simulink model "Quadcopter_v4_full"  (R2021a)
settings: Solver=ode4  StartTime=0.0  StopTime=87  FixedStep=0.001  RelTol=1e-6
values from neighbouring files (symbols this model uses):
  mean_wind = [2.72 , 1.75, -0.006]    [main_run.m]    (also in main_run_5_1.m; param_est.m = [2.72 , 1.75, .006])
  q = X(7:10)    [EKF_without_wind.m]
  r = linspace(floor(nr*0.01)/nr,1,nr)    [main_run.m]    (also in main_run_5_1.m)
  w1 = w(1)    [EKF_without_wind.m]
  x0 = [0,0,0,1,0,0,0,-P.mean_wind,0,0,0]    [main_run.m]    (also in main_run_5_1.m)
  xref = [1,1,-8,1,0,0,0,-P.mean_wind]    [main_run.m]    (also in main_run_5_1.m)
undefined symbols (not defined in the file or in its folder): HDBK, MIL, Moderate, P, u1, v1
libraries: simulink x1, aerolibwind2 x1
(part 5 of 5)

== matlab function Quadcopter_v4_full/Rotor Dynamics /SBEMT/Simplified BEMT ==
  data: V_rb input; Y output; rpm input; P parameter
function Y  = simplified_BEMT(V_rb,rpm,P)
%simplified BEMT model Summary of this function goes here
%   Detailed explanation goes here
% q_i  = X(4:7);
% vr_i = X(8:10);
% 
% eul = quat2eul(q_i')';
% eul([1 3]) = eul([3 1]);
% roll = eul(1);
% pitch = eul(2);
% yaw = eul(3);
% x_axis=[1;0;0];y_axis=[0;1;0];z_axis=[0;0;1]; 
% R_ib = expm(hat(z_axis)*yaw)*expm(hat(y_axis)*pitch)*expm(hat(x_axis)*roll);
% vr_b = R_ib'*vr_i;

% Asma: So Vr_b here is the exact input going into actual BMET optimization
% block, it is already calculated so no need for additional calculation
vr_b = V_rb;
rpm =mean(rpm)/16000;
%%
weights = P.weights;
n_lay_neu = P.n_lay_neu;

features = 4;
weights1 = cell(1,length(n_lay_neu));
for i=1:1:length(n_lay_neu)
    if i==1 
        index_input = features+1;                %+1 means add the bias row
        index_output = n_lay_neu(i);
        weights1{i} = weights(1:index_input,1:index_output);
    else
        index_input_pre = index_input;
        index_input = index_input_pre + n_lay_neu(i-1) + 1;
        index_output = n_lay_neu(i);
        weights1{i} = weights(index_input_pre+1:index_input,1:index_output);
    end 
end
%% 
% In order to require the code generator's requirement, we declare the
% thrust_forward_NN as the extrinsic function
coder.extrinsic('thrust_forward_NN'); 
Y = zeros(1);
Y = thrust_forward_NN([vr_b' rpm],weights1,n_lay_neu);%normalize the rpm(16000)
Y = 4*Y;
end

== matlab function Quadcopter_v4_full/wind/Dryden Wind/Input/DCM//rotation matrix ==
  data: x input; R output
function R = fcn(x)
phi = x(7);theta = x(8);psi = x(9);
% rotation from inertial frame to body frame
R = [1, 0, 0;0, cos(phi), sin(phi);0, -sin(phi), cos(phi)]*[cos(theta),...
    0, -sin(theta);0, 1, 0;sin(theta), 0, cos(theta)]*[cos(psi),...
    sin(psi), 0;-sin(psi), cos(psi), 0;0, 0, 1];
R = inv(R);
end

== matlab function Quadcopter_v4_full/wind/Dryden Wind/Input/MATLAB Function ==
  data: wind input; V output; vel input
function V = fcn(wind,vel)
%#codegen
V = norm(wind - vel);
end

== matlab function Quadcopter_v4_full/wind/Dryden Wind/Input1/DCM//rotation matrix ==
  data: x input; y output
function y = fcn(x)
phi = x(7);theta = x(8);psi = x(9);
% rotation from inertial frame to body frame
R = [1, 0, 0;0, cos(phi), sin(phi);0, -sin(phi), cos(phi)]*[cos(theta),...
    0, -sin(theta);0, 1, 0;sin(theta), 0, cos(theta)]*[cos(psi),...
    sin(psi), 0;-sin(psi), cos(psi), 0;0, 0, 1];
R = inv(R);
y = R;

== matlab function Quadcopter_v4_full/wind/Dryden Wind/Input1/MATLAB Function ==
  data: wind input; V output; vel input; P parameter
function V = fcn(wind,vel,P)
%#codegen
V = norm(wind - vel);
end

== matlab function Quadcopter_v4_full/wind/Dryden Wind/Select velocities/Merge Subsystems/convert to inertial frame ==
  data: ug input; ugw output; vg input; wg input; dcm input; vgw output; wgw output
function [ugw,vgw,wgw] = fcn(ug,vg,wg,dcm)
%#codegen
u = dcm*[ug;vg;wg];
ugw = u(1);
vgw = u(2);
wgw = u(3);

== matlab function Quadcopter_v4_full/quadcopter/MATLAB Function ==
  settings: updateMethod=DISCRETE
  data: X input; U input; wind input; t_c input; X_dot output; P parameter; wdot output; R output
function [X_dot,wdot,R]  = quad_model(X,U,wind,t_c,P)

%#codegen
%References: Dynamics using Quaternion for full-state feedback control
%adapted from "Onboard State Dependent LQR for Agile Quadrotors"
%see "AIAA paper draft for full model"

%parameters
m = P.m;
g = P.g;
rho = P.rho;

Ix = P.Ix;
Iy = P.Iy;
Iz = P.Iz;
J=[Ix , 0 , 0;
    0 , Iy , 0;
    0 , 0  , Iz];

D   = P.D;
%states
% p_i = X(1:3);
q_i  = X(4:7);
% hao 10/27/2021 normalize the unit quaternion
q_i=q_i/norm(q_i);

v_i = X(8:10);
w_b = X(11:13);
% disp(w_b)


%inputs

F_c = [0;0;U(1)];
tau=[U(2);
     U(3);
     U(4)];
 
%% system dynamics with drag in WORLD FRAME
%HAO: what is this?
% wind(3)=-wind(3);%wind from CFD data is positive upward

R=quater_rot(q_i);

% eul = quat2eul(q_i')';
% eul([1 3]) = eul([3 1]);
% roll = eul(1);
% pitch = eul(2);
% yaw = eul(3);
% x_axis=[1;0;0];y_axis=[0;1;0];z_axis=[0;0;1]; 
% R = expm(hat(z_axis)*yaw)*expm(hat(y_axis)*pitch)*expm(hat(x_axis)*roll);

% R = quat2R(q_i');



dp = v_i+wind;
dq = 0.5*quater_mult(q_i)*[0;w_b];
% dv = ([0;0;g] - R*F_c-norm(v_i)*R*D*R'*v_i)/m;
% dv = ([0;0;m*g] - R*F_c-0.5*rho*norm(v_i)*R*D*R'*v_i)/m; %10/20/2021 Hao
f_vr=-(1/2)*rho*D*norm(R'*v_i)*(R'*v_i);
dv = ([0;0;m*g] - R*F_c + R*f_vr)/m;


dwb = J\(tau-cross(w_b,(J*w_b)));

X_dot=[dp ; dq ; dv ; dwb]';
wdot=dwb;


end


function R = quater_rot(q)

w = q(1);
x = q(2);
y = q(3);
z = q(4);

Q = [w -x -y -z;...
     x w -z y;...
     y z w -x;...
     z -y x w];

Qc =[w -x -y -z;...
     x w z -y;...
     y -z w x;...
     z y -x w];
t = Qc'*Q;
R = t(2:4,2:4);
end


function Q = quater_mult(q)

w = q(1);
x = q(2);
y = q(3);
z = q(4);

Q = [w -x -y -z;...
     x w -z y;...
     y z w -x;...
     z -y x w];

end

== matlab function Quadcopter_v4_full/Controller /High Level Controller/trajectory/MATLAB Function ==
  data: t input; xdes output; P parameter
function xdes = getref(t,P)

% This function tracks time and match nominal trajectory at next nearest
% time
% Input:
% nomTraj is the nominal trajectory with t
% 
nomTraj = P.nomTraj;
idxA = find(nomTraj(:,1)>=t);
idx=idxA(1);
xdes=nomTraj(idx,2:end);

== matlab function Quadcopter_v4_full/MATLAB Function ==
  data: u input; omega output; P parameter
function omega = motor_omega(u, P)

%omega = u;
%prevent negative F because the calculation only need the value of fc
% if u(1)<0
%     u(1)=-u(1);
% end
%prevent too high of a moment
for i=2:3
    if u(i)>.15*u(1)
        u(i)=.15*u(1);    %why?
    end
end

L = P.l;
b= P.b;
k = P.k;
% 
A = [b b b b;
    0 L*b 0 -L*b;
    L*b 0 -L*b 0;   %from BMET Code 
    k -k k -k];  %

% A = [b b b b;
%     0 -L*b 0 L*b;
%     -L*b 0 L*b 0;   %from source Trajectory tracking control design with command-filtered compensation for a quadrotor
%     -k k -k k]; 


% A = [b b b b;
%     0 -L*b 0 L*b;
%     L*b 0 -L*b 0;   %Tryng my ways
%     k -k k -k];  %

%R matrix just changes which direction the 'front' of the quad is
%without it,quadcopter would be '+' type;with it,quadcopter would be 'x' type
% offset = pi/4;
% R = [1 0 0 0;
%     0 cos(offset) -sin(offset) 0;
%     0 sin(offset) cos(offset) 0;
%     0 0 0 1];
% omega_squared = pinv(A)*R*u; %pinv-Pseudoinverse

omega_squared = pinv(A)*u'; %pinv-Pseudoinverse

for i=1:4
    if omega_squared(i) < 0
        omega_squared(i) = 0;
    end
end

omega = sqrt(omega_squared);
%hao 20/27/2021 set limit to the rpm
% for i=1:4
%     if omega(i) >16000
%         omega(i) = 16000;
%     end
% end 

end

== matlab function Quadcopter_v4_full/Rotor Dynamics /BEMT(from datagen)/MATLAB Function1 ==
  settings: updateMethod=DISCRETE
  data: rpm_guesses input; V_rel_b input; U_final output; P parameter; geometry data_store_memory
function U_final  = FWF_BEMT_adjustment(rpm_guesses,V_rel_b, P)


% governing equations
% governing equations

% T=T1+T2+T3+T4 ;
% TA1=l*(T4-T2) ;   roll positive right wing down
% TA2=l*(T1-T3) ;   pitch up positive
% TA3=ta1+ta2+ta3+ta4 ;

% it looks like in atitude control output of the functin should be pitch
% down positive
% Not Related with LQR CONTROL ASMA*

%%
% predefining vriables for Codegen

k = P.k;
b = P.b;
l = P.l;
T_final=0;
Tau_initial=zeros(3,1);
Tau_final=zeros(3,1);
T2=zeros(4,1);
pow=zeros(4,1);

TA=zeros(3,1);
TA1=zeros(4,1);
TA2=zeros(4,1);
TA3=zeros(4,1);
ta1=zeros(4,1);
ta2=zeros(4,1);
ta3=zeros(4,1);

RPM2=single(zeros(4,1));
RPM=zeros(4,1);

T = b * rpm_guesses.^2;       % requested thrust from rotor r
Tau = k * rpm_guesses.^2;     % requested torques from rotor r

%%for calculation transforming all information into vector form
% rel_speed = V_info(1);
% heading = deg2rad(V_info(2));
% v_rel_z = V_info(3);
% 
% v_rel_x = rel_speed*cos(heading);
% v_rel_y = rel_speed*sin(heading);
% 
% V_rel_b = [v_rel_x,v_rel_y,v_rel_z];


for i=1:4
    % optimization to find optimum rpm where both momentum annd blade element theories match
    
    subfcn2 = @(rpm) try1(rpm,V_rel_b,T(i));
    
    rpm=golden_search(0,17000,subfcn2); %limits of RPM, checked that the higher limit goes beyond 25000 so chaging from 100 16000
    
    [~,roll,pitch,yaw,~,lambda1]=try1(rpm,V_rel_b,T(i));
    
    % rpm to rad/second
    RPM(i)=rpm ;%*2*pi/60; NO NEED ASMA
    
    % torques of a rotor - rotor 1 is the leading edge rotor,left
    % number 2, right number 4, aft number, 1 and 3 ccw. 2 and 4 cw.
    
    heading=atan(V_rel_b(2)/(V_rel_b(1)+0.000001));
    ta1(i) = roll * cos(heading) * (-1)^(i+1) - pitch * sin(heading);
    ta2(i) = roll * sin(heading) * (-1)^(i+1) + pitch * cos(heading) ;
    % the sign will be taken care of in Matrix M -- no worries!
    ta3(i) = yaw * (+1)^(i+1); %??? ASMA
    
end

Tau_initial=[sum(ta1);sum(ta2);sum(ta3)];

%% new addition to help with yaw moment

% here we need to find a way to change RPMs a bit such that they also
% provide the required Ta3. So, we can find the thrust and torque
% coefficients for a specific time and flight condition.

bb=T./RPM.^2;
kk=ta3./RPM.^2;

M=[bb'; ...
  0,bb(2)*l,0,-bb(4)*l;...
  bb(1)*l,0,-bb(3)*l,0;...
  kk(1),-kk(2),kk(3),-kk(4)];

% M=double([bb'; ...
%   0,-bb(2)*l,0,bb(4)*l;...
%   bb(1)*l,0,-bb(3),0;...
%   kk(1),-kk(2),kk(3),-kk(4)]);  %ASMA

T_tot=sum(T);

% we use the requsted thrust and torque - here we used the actual
% conventions, down pos z, right wing pos y, pointing to nose pos x
TA(1) = l* (T(2)-T(4)) - Tau_initial(1); % roll
TA(2) = l* (T(1)-T(3)) - Tau_initial(2); % pitch
TA(3) = dot([k,-k,k,-k],rpm_guesses.^2'); % yaw



%ASMA
%  TA(1) = l* (T(4)-T(2)) - Tau_initial(1); % roll
% TA(2) = l* (T(1)-T(3)) - Tau_initial(2); % pitch
% TA(3) = dot([-k,k,-k,k],rpm_guesses.^2'); % yaw

u_temp= [T_tot;TA(1);TA(2);TA(3)];
% newly obtained RPMs Original
% RPM2=(M\[T_tot;TA(1);TA(2);TA(3)]).^0.5;

%%ADDED BY ASMA
RPM_SQ = pinv(M)*u_temp;

for i=1:4
    if RPM_SQ(i) < 0
        RPM_SQ(i) = 0;
    end
end

RPM2 = sqrt(RPM_SQ);

% now let's see how much thrust and torque they make

for i=1:4
    % input to propeller code must be RPM not rev/sec
    
    subfcn2 = @(T) try2(T,rpm,V_rel_b);
    
    T=golden_search(0,40,subfcn2);  %THIS IS FOR THURST
    
    [~,roll,pitch,yaw,T,lambda2]=try2(T,rpm_guesses(i),V_rel_b);
    pow(i)=yaw * RPM2(i);
    T2(i)=T;
    heading=atan(V_rel_b(2)/(V_rel_b(1)+0.000001));
    TA1(i) = roll * cos(heading) * (-1)^(i+1) - pitch * sin(heading);
    TA2(i) = roll * sin(heading) * (-1)^(i+1) + pitch * cos(heading) ;
    TA3(i)=yaw* (-1)^(i+1);
end

TA_rotor=[sum(TA1);sum(TA2);sum(TA3)];

% here since we don't use negative thrusts, conventions are changed
T_final=sum(T2);
Tau_final(1,1)=l*(T2(2)-T2(4))+TA_rotor(1) ; % roll
Tau_final(2,1)=l*(T2(1)-T2(3))+ TA_rotor(2) ; % pitch
Tau_final(3,1)=TA_rotor(3) ;

%ASMA
%  Tau_final(1,1)=l*(T2(4)-T2(2))+ TA_rotor(1) ; % roll 

power = sum(pow) ;

U_final=[T_final,Tau_final'];
local_param= [bb , kk];
end

== matlab function Quadcopter_v4_full/wind/sinusoidal_wind/sinusoidal part ==
  data: LES input; y output; t input
function y = fcn(LES,t)
ux=2.7;
uy=1.7;
uz=0;
dx = LES(1) - ux + 3*sin(2*pi*(1/50)*t); 
dy = LES(2) - uy + 2*sin(2*pi*(1/50)*t); 
dz = LES(3) - uz + 0.5*sin(2*pi*(1/50)*t); 
y = [dx;dy;dz];

== matlab function Quadcopter_v4_full/quadcopter/initial states/MATLAB Function1 ==
  data: X0 output
function X0  = fcn()
% X0 = [10*randn;10*randn;10*randn;2*randn;2*randn;2*randn;...
%      (pi/4)*randn;(pi/4)*randn;(pi/4)*randn;0;0;0;];
X0 = [10*randn;10*randn;10*randn;1*randn;1*randn;1*randn;...
     0.1*randn;0.1*randn;0.1*randn;0.1*randn;0.1*randn;0.1*randn];
end

== matlab function Quadcopter_v4_full/Estimator/Estimator/states_aug ==
  data: accel_gyro input; states input; states_aug output
function states_aug = fcn(accel_gyro,states)
%states for Asma's controller
gyro = accel_gyro(4:6);
states_aug = [states;gyro];

== matlab function Quadcopter_v4_full/Rotor Dynamics /BEMT/BEMT Adjustment ==
  settings: updateMethod=DISCRETE
  data: rpm_guesses input; RPM output; V_rel_b input; P parameter; RPM2 output; Tau_initial output; Tau_final output; power output; T_final output; U_final output; geometry data_store_memory; local_param output
function [RPM,RPM2,Tau_initial,Tau_final,power,T_final,U_final,local_param] = FWF(rpm_guesses,V_rel_b, P)


% governing equations
% governing equations

% T=T1+T2+T3+T4 ;
% TA1=l*(T4-T2) ;   roll positive right wing down
% TA2=l*(T1-T3) ;   pitch up positive
% TA3=ta1+ta2+ta3+ta4 ;

% it looks like in atitude control output of the functin should be pitch
% down positive
% Not Related with LQR CONTROL ASMA*

%%
% predefining vriables for Codegen

k = P.k;
b = P.b;
l = P.l;
T_final=0;
Tau_initial=zeros(3,1);
Tau_final=zeros(3,1);
T2=zeros(4,1);
pow=zeros(4,1);

TA=zeros(3,1);
TA1=zeros(4,1);
TA2=zeros(4,1);
TA3=zeros(4,1);
ta1=zeros(4,1);
ta2=zeros(4,1);
ta3=zeros(4,1);

% RPM2=single(zeros(4,1));
RPM2=zeros(4,1);
RPM=zeros(4,1);

T = b * rpm_guesses.^2;       % requested thrust from rotor r
Tau = k * rpm_guesses.^2;     % requested torques from rotor r

for i=1:4
    % optimization to find optimum rpm where both momentum annd blade element theories match
    
    subfcn2 = @(rpm) try1(rpm,V_rel_b,T(i));
    
%     rpm=golden_search(0,25000,subfcn2); %limits of RPM, checked that the higher limit goes beyond 25000 so chaging from 100 16000
    rpm=golden_search(0,17000,subfcn2); % HAO the 17000 is to keep consistent with BEMT in datagen 
    [~,roll,pitch,yaw]=try1(rpm,V_rel_b,T(i));
    
    % rpm to rad/second
    RPM(i)=rpm ;%*2*pi/60; NO NEED ASMA
    
    % torques of a rotor - rotor 1 is the leading edge rotor,left
    % number 2, right number 4, aft number, 1 and 3 ccw. 2 and 4 cw.
    
    heading=atan(V_rel_b(2)/(V_rel_b(1)+0.000001));
    ta1(i) = roll * cos(heading) * (-1)^(i+1) - pitch * sin(heading);
    ta2(i) = roll * sin(heading) * (-1)^(i+1) + pitch * cos(heading) ;
    % the sign will be taken care of in Matrix M -- no worries!
    ta3(i) = yaw * (+1)^(i+1); %??? ASMA
    
end

Tau_initial=[sum(ta1);sum(ta2);sum(ta3)];

%% new addition to help with yaw moment

% here we need to find a way to change RPMs a bit such that they also
% provide the required Ta3. So, we can find the thrust and torque
% coefficients for a specific time and flight condition.

bb=T./RPM.^2;
kk=ta3./RPM.^2;

M=[bb'; ...
  0,bb(2)*l,0,-bb(4)*l;...
  bb(1)*l,0,-bb(3)*l,0;...
  kk(1),-kk(2),kk(3),-kk(4)];

% M=double([bb'; ...
%   0,-bb(2)*l,0,bb(4)*l;...
%   bb(1)*l,0,-bb(3),0;...
%   kk(1),-kk(2),kk(3),-kk(4)]);  %ASMA

T_tot=sum(T);

% we use the requsted thrust and torque - here we used the actual
% conventions, down pos z, right wing pos y, pointing to nose pos x
TA(1) = l* (T(2)-T(4)) - Tau_initial(1); % roll
TA(2) = l* (T(1)-T(3)) - Tau_initial(2); % pitch
TA(3) = dot([k,-k,k,-k],rpm_guesses.^2'); % yaw



%ASMA
%  TA(1) = l* (T(4)-T(2)) - Tau_initial(1); % roll
% TA(2) = l* (T(1)-T(3)) - Tau_initial(2); % pitch
% TA(3) = dot([-k,k,-k,k],rpm_guesses.^2'); % yaw

u_temp= [T_tot;TA(1);TA(2);TA(3)];
% newly obtained RPMs Original
% RPM2=(M\[T_tot;TA(1);TA(2);TA(3)]).^0.5;

%%ADDED BY ASMA
RPM_SQ = pinv(M)*u_temp;

for i=1:4
    if RPM_SQ(i) < 0
        RPM_SQ(i) = 0;
    end
end

RPM2 = sqrt(RPM_SQ);

% now let's see how much thrust and torque they make

for i=1:4
    % input to propeller code must be RPM not rev/sec
    
    subfcn2 = @(T) try2(T,rpm,V_rel_b);
    
    T=golden_search(0,40,subfcn2);  %THIS IS FOR THURST
    
%     [~,roll,pitch,yaw,T]=try2(T,RPM2(i),V_rel_b);
    [~,roll,pitch,yaw,T]=try2(T,rpm_guesses(i),V_rel_b); % HAO the argument in here is to keep consistent with BEMT in datagen 
    pow(i)=yaw * RPM2(i);
    T2(i)=T;
    heading=atan(V_rel_b(2)/(V_rel_b(1)+0.000001));
    TA1(i) = roll * cos(heading) * (-1)^(i+1) - pitch * sin(heading);
    TA2(i) = roll * sin(heading) * (-1)^(i+1) + pitch * cos(heading) ;
    TA3(i)=yaw* (-1)^(i+1);
end

TA_rotor=[sum(TA1);sum(TA2);sum(TA3)];

% here since we don't use negative thrusts, conventions are changed
T_final=sum(T2);
Tau_final(1,1)=l*(T2(2)-T2(4))+TA_rotor(1) ; % roll
Tau_final(2,1)=l*(T2(1)-T2(3))+ TA_rotor(2) ; % pitch
Tau_final(3,1)=TA_rotor(3) ;

%ASMA
%  Tau_final(1,1)=l*(T2(4)-T2(2))+ TA_rotor(1) ; % roll 

power = sum(pow) ;

U_final=[T_final,Tau_final'];
local_param= [bb , kk];
end
